simulink model "MotorControl_2"  (Simulink 8.1)
settings: Solver=FixedStepDiscrete  StartTime=0.0  StopTime=20  FixedStep=0.5  RelTol=1e-3
PostLoadFcn:
  | MotorControl_2_data
undefined symbols (not defined in the file or in its folder): A14, B, B13, D, L3, R10
libraries: BAMLIB564xL x5, rappid_564xl_ec_toolbox x1
settings Model: Creator=evarshavskaya  LastModifiedBy=evarshavskaya
settings DataIOCC: ExternalInput=off  InitialState=off  SaveOutput=off  SignalLogging=off  SaveTime=off
settings OptimizationCC: InlineParams=on  OptimizeModelRefInitCode=on  LifeSpan=1
settings DebuggingCC: InheritedTsInSrcMsg=none  SingleTaskRateTransMsg=error  ParameterPrecisionLossMsg=none  UnconnectedInputMsg=error  UnconnectedOutputMsg=error  UnconnectedLineMsg=error  UnknownTsInhSupMsg=error
settings HardwareCC: ProdLargestAtomicInteger=Long  ProdLargestAtomicFloat=Double  ProdIntDivRoundTo=Zero  ProdEndianess=BigEndian  ProdHWDeviceType=Freescale->32-bit PowerPC
settings RTWCC: SystemTargetFile=rappid564xl.tlc  MakeCommand=rappid_564xl_make_rtw  TemplateMakefile=rappid_564xl_default_tmf  PostCodeGenCommand=rappid_analyzegencode(buildInfo)  Description=RAppID Toolbox MPC564xL Code Generation Target (rappid)  ProcessScript=rappid564xl_make_rtw_hook
settings CodeAppCC: IgnoreCustomStorageClasses=off  CustomSymbolStrType=$N$R$M  InternalIdentifier=Classic
settings STFCustomTargetCC: CodeReplacementLibrary=ANSI_C  ModelReferenceCompliant=off  CombineOutputUpdateFcns=on  SuppressErrorStatus=on  ERTCustomFileBanners=on  SupportContinuousTime=off  SupportNonInlinedSFcns=off  MATLABClassNameForMDSCustomization=Simulink.SoftwareTarget.ERTCustomization  GRTInterface=off  SystemTargetFile=rappid564xl.tlc
settings ERTTargetCC: CodeReplacementLibrary=ANSI_C  MultiwordLength=2048  ModelReferenceCompliant=off  ParMdlRefBuildCompliant=off  CompOptLevelCompliant=off  ConcurrentExecutionCompliant=off  SuppressErrorStatus=on  ERTFirstTimeCompliant=off  ModelStepFunctionPrototypeControlCompliant=off  CPPClassGenCompliant=off  ExtModeMexFile=noextcomm  InlinedParameterPlacement=NonHierarchical  ERTCustomFileTemplate=example_file_process.tlc  ConvertIfToSwitch=off  SuppressUnreachableDefaultCases=off

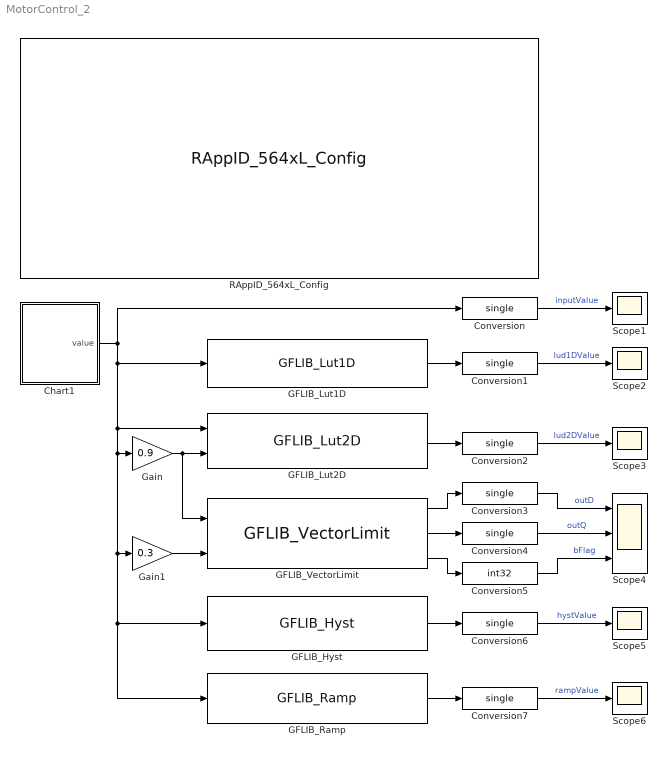
== system MotorControl_2 ==
  Chart1 : Stateflow chart  TreatAsAtomicUnit=on
  Conversion{,1..4,6..7} (7 alike) : DataTypeConversion  OutDataTypeStr=single
  Conversion5 : DataTypeConversion  OutDataTypeStr=int32
  GFLIB_Hyst : BAMLIB564xL/General Functions/GFLIB_Hyst  s32HystOn=s32HystOn  s32HystOff=s32HystOff  s32OutValOn=s32OutValOn  s32OutValOff=s32OutValOff
  GFLIB_Lut1D : BAMLIB564xL/General Functions/GFLIB_Lut1D  s32ShamOffset=s32ShamOffset  ps32Table=ps32Table  s32MidIdx=s32MidIdx
  GFLIB_Lut2D : BAMLIB564xL/General Functions/GFLIB_Lut2D  s32ShamOffset1=s32ShamOffset1  s32ShamOffset2=s32ShamOffset2  ps32Table=ps32Table2  s32MidId=s32MidIdx2
  GFLIB_Ramp : BAMLIB564xL/General Functions/GFLIB_Ramp  s32RampUp=s32RampUp  s32RampDown=s32RampDown
  GFLIB_VectorLimit : BAMLIB564xL/General Functions/GFLIB_VectorLimit  s32Lim=s32Lim
  Gain : Gain  Gain=0.9  OutDataTypeStr=single
  Gain1 : Gain  Gain=0.3  OutDataTypeStr=single
  RAppID_564xL_Config : rappid_564xl_ec_toolbox/MPC564xL/RAppID_564xL_Config  SystemClock=120  XTAL=40  MC_clock_60=12  MC_clock_80=16  MC_clock_120=10  SWG_clock_60=20  SWG_clock_80=13.334  SWG_clock_120=20  Compiler=CodeWarrior  MemTarget=RAM  Part=MPC5643L  Package=144 LQFP  global_int_priority=10  base_tick_priority=14  sys_task_supress=off  exception_handlers=off  stored_mdl_name=MotorControl_2  freemaster_interface=Oops  freemaster_rx_pin="LINFlex_0 Rx Pin 116 : \"PB[3]\""  freemaster_tx_pin="LINFlex_0 Tx Pin 114 : \"PB[2]\""  freemaster_interface_1=Serial 0  freemaster_enable=on  freemaster_rate=57600  freemaster_tx0_pin=18 : B[2] : 114 : A14  freemaster_rx0_pin=19 : B[3] : 116 : B13  freemaster_tx1_pin=57 : D[9] : 26 : L3  freemaster_rx1_pin=29 : B[13] : 60 : R10  freemaster_can_channel=1CH  freemater_can_speed=500K  freemaster_can_msgig=0x7AA  ccp_interface=None  ccp_enable=off  ccp_can_channel=CH1 (MB 0 - 1)  ccp_can_speed=500K  ccp_can_cro_id=256  ccp_can_dto_id=257  ccp_dev_id=RappID  ccp_dev_addr=0  ccp_odt=3  ccp_daq=3  pil_enable=off  pil_bam=on  comport=1  pil_rate=57600  bam_password_def=on  bam_password=0xFEEDFACECAFEBEEF  bam_sa_cs=off  bam_start_address=0x0  bam_code_size=0x7000  cons_dspi=on  cons_can=on  cons_adc=on  cons_pwm=on  cons_ctu=on  cons_swg=on  cons_eTimer=on  cons_fm=on
  Scope{1..3,5..6} (5 alike) : Scope
      Scope1 settings: TickLabels=on  TimeRange=20  YMin=0  YMax=1
      Scope2 settings: TickLabels=on  TimeRange=20  YMin=0  YMax=1
      Scope3 settings: TickLabels=on  TimeRange=20  YMin=0  YMax=1  SaveName=ScopeData2
      Scope5 settings: TickLabels=on  TimeRange=20  YMin=0  YMax=1  SaveName=ScopeData4
      Scope6 settings: TickLabels=on  TimeRange=20  YMin=0  YMax=1  SaveName=ScopeData5
  Scope4 : Scope  NumInputPorts=3
      settings: TickLabels=on  TimeRange=20  YMin=0~0~0  YMax=1~1~1  SaveName=ScopeData3
  wires:
  Chart1/1(value) -> GFLIB_Lut1D/1, Gain/1, Gain1/1, GFLIB_Hyst/1, GFLIB_Ramp/1, GFLIB_Lut2D/1, Conversion/1
  GFLIB_Lut1D/1 -> Conversion1/1
  GFLIB_Lut2D/1 -> Conversion2/1
  Gain/1 -> GFLIB_Lut2D/2, GFLIB_VectorLimit/1
  Gain1/1 -> GFLIB_VectorLimit/2
  GFLIB_VectorLimit/1 -> Conversion3/1
  GFLIB_VectorLimit/2 -> Conversion4/1
  GFLIB_VectorLimit/3 -> Conversion5/1
  GFLIB_Hyst/1 -> Conversion6/1
  GFLIB_Ramp/1 -> Conversion7/1
  Conversion/1 -> Scope1/1  "inputValue"
  Conversion1/1 -> Scope2/1  "lud1DValue"
  Conversion2/1 -> Scope3/1  "lud2DValue"
  Conversion4/1 -> Scope4/2  "outQ"
  Conversion3/1 -> Scope4/1  "outD"
  Conversion5/1 -> Scope4/3  "bFlag"
  Conversion6/1 -> Scope5/1  "hystValue"
  Conversion7/1 -> Scope6/1  "rampValue"

== stateflow chart Chart1 ==
  settings: executeAtInitialization=1
  state A
    du:
    value=cntr;
    cntr=cntr+0.05;
    ex:
    cntr = 0;
  (default) -> A : {cntr=0;}
  A -> A : [cntr >= 1]
  data: cntr local single [0..2] =0; value output single [0..2]
